simulink model "sedemo_rngseeds_mgmt"  (Simulink 7.5)
settings: Solver=VariableStepDiscrete  StartTime=0.0  StopTime=10.0  RelTol=1e-3
libraries: simeventssink1 x2, simeventsgenerators1 x2, simeventsqueue1 x1, simeventsinfo x1, simeventsrouting1 x1, simeventsattributes2 x1
settings Model: Creator=The MathWorks Inc.
settings OptimizationCC: InitFltsAndDblsToZero=on
settings DebuggingCC: SolverPrmCheckMsg=none  StrictBusMsg=Warning
settings SimEventsCC: propDiagAttribOutput=1  propDiagFcnCallOutput=1  propDiagStatOutput=0

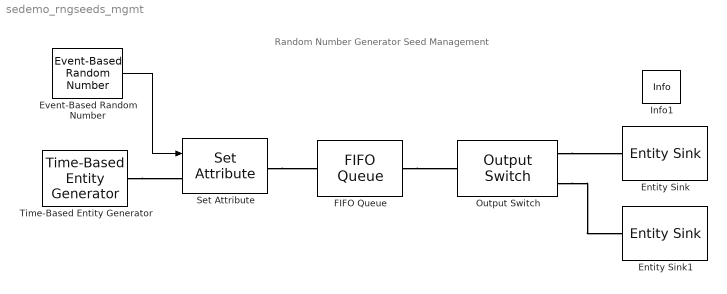
== system sedemo_rngseeds_mgmt ==
  note: Random Number Generator Seed Management
  Entity Sink : simeventssink1/Entity Sink  Priority=1  SystemSampleTime=-1  AvailableForArrivals=on  StatNumberArrived=Off
  Entity Sink1 : simeventssink1/Entity Sink  Priority=1  SystemSampleTime=-1  AvailableForArrivals=on  StatNumberArrived=Off
  Event-Based Random Number : simeventsgenerators1/Signal Generators/Event-Based Random Number  SystemSampleTime=-1  distribution=Uniform  meanExp=1  minUnif=0  maxUnif=1  pOneBern=0.25  pSuccessBino=0.5  numTrialBino=1  meanNorm=0  stdNorm=1  minTri=1  maxTri=3  modeTri=2  thresholdLogn=0  scaleLogn=1  shapeLogn=1  pSuccessGeo=0.5  meanPoiss=1  thresholdLogl=0  scaleLogl=1  thresholdGam=0  scaleGam=1  shapeGam=1  minBeta=0  maxBeta=1  shape1Beta=1  shape2Beta=1  minUnid=0  maxUnid=1  numValueUnid=2  thresholdWbl=0  scaleWbl=1  shapeWbl=1  valueVecCont=[0 1]  cdfVecCont=[0 1]  valueVecDisc=[0 1]  probVecDisc=[0.5 0.5]  seed=12345  IsProcessed=on  isConnected=1
  FIFO Queue : simeventsqueue1/FIFO Queue  Priority=1  SystemSampleTime=-1  Capacity=25  EnableTOPort=off  StatNumberDeparted=Off  StatNumberInBlock=Off  StatPendingEntity=Off  StatAverageWait=Off  StatAverageQueueLength=Off  StatNumberTimedout=Off
  Info1 : simeventsinfo/Info  SystemSampleTime=-1
  Output Switch : simeventsrouting1/Output Switch  Priority=1  SystemSampleTime=-1  NumberOutputPorts=2  SwitchingCriterion=Equiprobable  InitialSeed=12345  AttributeName=Attribute1  InitialConditionsOpt=off  InitialConditions=1  EntityBufferOpt=off  SpecifyEventPriority=off  PriorityOutputSwitchSelectPort=4100  TimeoutPortOpt=off  StatNumberDeparted=Off  StatNumberTimedOut=Off  StatPendingEntity=Off  StatLastDeparturePort=Off  EvaluatedNumPorts=2
  Set Attribute : simeventsattributes2/Set Attribute  Priority=1  DialogController=des_ddg_create  DialogControllerArgs=DataTag5  SystemSampleTime=-1  AttributeFrom=Signal port  AttributeName=Attribute1  AttributeTreatAsVector=1  AttributeValue=1  AttributeCreate=on  StatNumberDeparted=Off  EvaluatedAttributeValue={[]}
  Time-Based Entity Generator : simeventsgenerators1/Entity Generators/Time-Based Entity Generator  Priority=1  DialogController=des_ddg_create  DialogControllerArgs=DataTag7  SystemSampleTime=-1  GenerateEntitiesUpon=Intergeneration time from dialog  Distribution=Uniform  Minimum=0  Maximum=1  Mean=1  InitialSeed=6548  Period=1  PriorityEntityGeneration=300  GenerateEntityAtSimulationStart=off  ResponseWhenBlocked=Pause generation  ResponseWhenUnblocked=Immediate restart  EntityType=Blank  StatNumberDeparted=Off  StatPendingEntity=Off  StatAverageIntergenerationTime=Off
  wires:
  Event-Based Random Number/1 -> Set Attribute/1
  connections:
  Time-Based Entity Generator/RConn1 -- Set Attribute/LConn1
  Output Switch/RConn1 -- Entity Sink/LConn1
  Output Switch/RConn2 -- Entity Sink1/LConn1
  Set Attribute/RConn1 -- FIFO Queue/LConn1
  FIFO Queue/RConn1 -- Output Switch/LConn1
